simulink model "untitled"  (R2021a)
settings: Solver=VariableStepAuto  StartTime=0.0  StopTime=inf  RelTol=1e-3
settings Model: Creator=surya  LastModifiedBy=surya

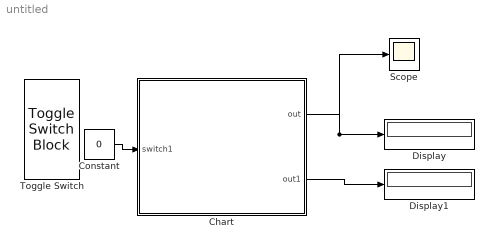
== system untitled ==
  Chart : Stateflow chart  TreatAsAtomicUnit=on
  Constant : Constant  Value=0
  Display : Display
  Display1 : Display
  Scope : Scope
  Toggle Switch : ToggleSwitchBlock
      settings: Values={{'Off', 'On'}, [0 1]}
  wires:
  Chart/1(out) -> Scope/1, Display/1
  Constant/1 -> Chart/1(switch1)
  Chart/2(out1) -> Display1/1

== stateflow chart untitled/Chart ==
  state counter1(y) [function]
    (default) -> (junction 21) : % counter to 500
    (junction 21) -> (junction 23) : {y1=y}
    (junction 23) -> (junction 22) [order 1] : [y1<500]
    (junction 24) -> (junction 23)
    (junction 22) -> (junction 24) : {y1=y1+1;}
    (junction 23) -> (junction 25) [order 2] : {out1=y1}
  state Fancontrol
    state FanOff
      en:out=0;
    state FanOn
      en:out=1;
    (junction 8) -> FanOn : [out1>=500]
    FanOff -> (junction 8) : [switch1==1]{counter1(0)}
    (default) -> FanOff
    FanOn -> FanOff : [switch1==0]{out1=0}
  data: y function_input; out output; switch1 input; out1 output
